simulink model "untitled2"  (R2013a)
settings: Solver=ode1  StartTime=0.0  StopTime=10.0  FixedStep=0.0001  RelTol=1e-3
settings Model: Creator=mohammad  LastModifiedBy=mohammad

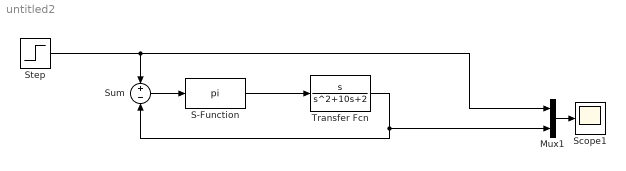
== system untitled2 ==
  Mux1 : Mux  Inputs=2
  S-Function : S-Function  FunctionName=pi  Parameters=0.0001,1,1  EnableBusSupport=off
  Scope1 : Scope
      settings: YMin=0.4  YMax=1.5
  Step : Step  Time=3  SampleTime=0
  Sum : Sum  Inputs=+-
  Transfer Fcn : TransferFcn  Numerator=[1 0]  Denominator=[1 10 2]
  wires:
  Transfer Fcn/1 -> Mux1/2, Sum/2
  S-Function/1 -> Transfer Fcn/1
  Sum/1 -> S-Function/1
  Mux1/1 -> Scope1/1
  Step/1 -> Mux1/1, Sum/1
